simulink subsystem "metszespont"  (R2024b)
settings: Solver=VariableStepAuto  StartTime=0.0  StopTime=10.0  RelTol=1e-3
settings Model: Creator=Asus  LastModifiedBy=Asus

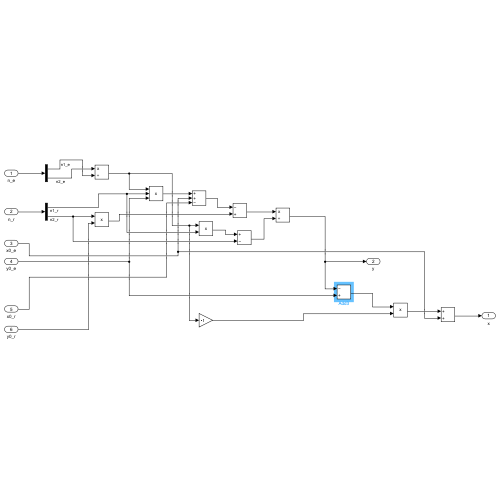
[thumbnail: Simulink's stored preview of the top-level diagram]
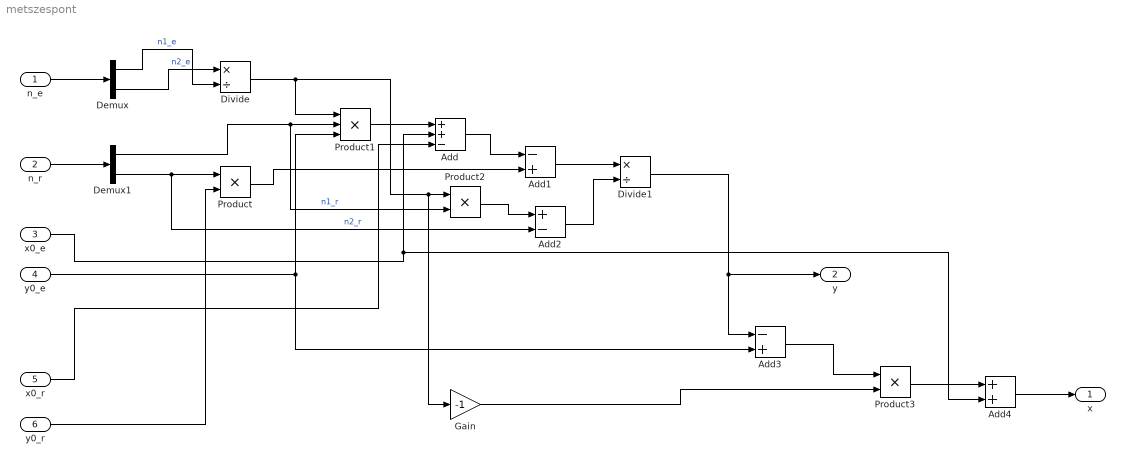
== system metszespont ==
  n_e : Inport
  n_r : Inport  Port=2
  x0_e : Inport  Port=3
  y0_e : Inport  Port=4
  x0_r : Inport  Port=5
  y0_r : Inport  Port=6
  Add : Sum  Inputs=++-
  Add1 : Sum  Inputs=-+
  Add2 : Sum  Inputs=+-
  Add3 : Sum  Inputs=-+
  Add4 : Sum
  Demux : Demux  Outputs=2
  Demux1 : Demux  Outputs=2
  Divide : Product  Inputs=*/
  Divide1 : Product  Inputs=*/
  Gain : Gain  Gain=-1
  Product : Product
  Product1 : Product  Inputs=3
  Product2 : Product
  Product3 : Product
  x : Outport
  y : Outport  Port=2
  wires:
  n_r/1 -> Demux1/1
  Demux1/1 -> Product2/2, Product1/2  "n1_r"
  Demux1/2 -> Add2/2, Product/1  "n2_r"
  Demux/1 -> Divide/2  "n1_e"
  Demux/2 -> Divide/1  "n2_e"
  y0_r/1 -> Product/2
  Divide/1 -> Product2/1, Gain/1, Product1/1
  y0_e/1 -> Add3/2, Product1/3
  x0_e/1 -> Add4/2, Add/2
  x0_r/1 -> Add/3
  Add/1 -> Add1/1
  Product/1 -> Add1/2
  Add1/1 -> Divide1/1
  Product1/1 -> Add/1
  Product2/1 -> Add2/1
  Add2/1 -> Divide1/2
  Divide1/1 -> Add3/1, y/1
  Add3/1 -> Product3/1
  Gain/1 -> Product3/2
  Product3/1 -> Add4/1
  Add4/1 -> x/1
  n_e/1 -> Demux/1
